simulink model "PubIfDecisionLSM_MDL"  (R2020b)
settings: configuration reference "DspaceConfig" (kept outside this file)
PostLoadFcn:
  | if any(exist('dsrtsu_mdlpostloadfcn', 'file') ~= 0), dsrtsu_mdlpostloadfcn('Execute', bdroot); end
InitFcn:
  | , if any(exist('rtifpga_mdlclblib', 'file') ~= 0), rtifpga_mdlclblib('Init', bdroot); end,
  | , if any(exist('dsmpb_private', 'file') ~= 0), dsmpb_private('dsmpb_mdlclblib', 'Init', bdroot); end,
values from neighbouring files (symbols this model uses):
  P_LSM_ALC_Enable = 0.0    [LSM_Parameter.sldd]
  P_LSM_AwayEdge_offset = 0.1    [LSM_Parameter.sldd]
  P_LSM_CentValidErr = 1.0    [LSM_Parameter.sldd]
  P_LSM_DOP_C0_EN_Limit = 0.8    [LSM_Parameter.sldd]
  P_LSM_DOP_C0_out_Limit = 2.0    [LSM_Parameter.sldd]
  P_LSM_DOP_C1_EN_Limit : value not decoded    [LSM_Parameter.sldd]
  P_LSM_DOP_C1_out_Limit : value not decoded    [LSM_Parameter.sldd]
  P_LSM_DOP_C1AndC2_Lim_X : value not decoded    [LSM_Parameter.sldd]
  P_LSM_DOP_C2_EN_Limit : value not decoded    [LSM_Parameter.sldd]
  P_LSM_DOP_C2_out_Limit : value not decoded    [LSM_Parameter.sldd]
  P_LSM_DOP_In_Pre2Dop_Dis = 1.0    [LSM_Parameter.sldd]
  P_LSM_DOP_Out_Pre2Dop_Dis = 2.0    [LSM_Parameter.sldd]
  P_LSM_DOP_PreDis_X : value not decoded    [LSM_Parameter.sldd]
  P_LSM_DOP_PreDis_Y : value not decoded    [LSM_Parameter.sldd]
  P_LSM_DOPEnableSW = 1.0    [LSM_Parameter.sldd]
  P_LSM_DOPValid_CheckTime = 0.06    [LSM_Parameter.sldd]
  P_LSM_DoubleLine_Curr2Cent_Dislimit = 0.5    [LSM_Parameter.sldd]
  P_LSM_DoubleLine_Dop2Cent_Dislimit = 0.5    [LSM_Parameter.sldd]
  P_LSM_DoubleLine_DOPOut_C1 : value not decoded    [LSM_Parameter.sldd]
  P_LSM_DoubleLine_Pre2Cent_Dislimit = 1.0    [LSM_Parameter.sldd]
  P_LSM_Error_Limit = 0.5    [LSM_Parameter.sldd]
  P_LSM_IFV2CenterAxis = 0.0    [LSM_Parameter.sldd]
  P_LSM_IFV2RearAxis = 0.0    [LSM_Parameter.sldd]
  P_LSM_Line2Edge_limit = 0.5    [LSM_Parameter.sldd]
  P_LSM_Line_Error = 0.1    [LSM_Parameter.sldd]
  P_LSM_LineSTD_Limit = 0.15    [LSM_Parameter.sldd]
  P_LSM_NOH_Switch = 0.0    [LSM_Parameter.sldd]
  P_LSM_OTL_C0_Factor = 1.0    [LSM_Parameter.sldd]
  P_LSM_OTL_C1_Factor = 0.5    [LSM_Parameter.sldd]
  P_LSM_OTL_C2_Factor = 0.5    [LSM_Parameter.sldd]
  P_LSM_Pre2OnlyLineDis = 5.0    [LSM_Parameter.sldd]
  P_LSM_Pre_t = 0.0    [LSM_Parameter.sldd]
  P_LSM_SingleLine_Cent2Edge_Dislimit = 100.0    [LSM_Parameter.sldd]
  P_LSM_SingleLine_Curr2Cent_Dislimit = 0.2    [LSM_Parameter.sldd]
  P_LSM_SingleLine_Dop2Cent_Dislimit = 0.2    [LSM_Parameter.sldd]
  P_LSM_SingleLine_DOPOut_C1 : value not decoded    [LSM_Parameter.sldd]
  P_LSM_SingleLine_Pre2Cent_Dislimit = 0.5    [LSM_Parameter.sldd]
  P_LSM_TJALimitSpd = 60.0    [LSM_Parameter.sldd]
undefined symbols (not defined in the file or in its folder): P_lCS_IFV2CenterAxis, P_LCS_IFV2RearAxis, P_LSM_EntryEdge_offset, P_LSM_EntryLnChngEnSwitch, P_LSM_EntryVanishDis, P_LSM_LinetLostTime, P_LSM_LineWijCal_C12, P_LSM_LineWijCal_C13, P_LSM_MapValid_ErrorSwitch, P_LSM_PosLineLcFac, P_LSM_SpdLim_Stub_Spd, P_LSM_SpdLim_StubLength, P_LSM_SpdTurnAlarm
libraries: simulink x324, TrueDurationTime x11
(part 7 of 25)

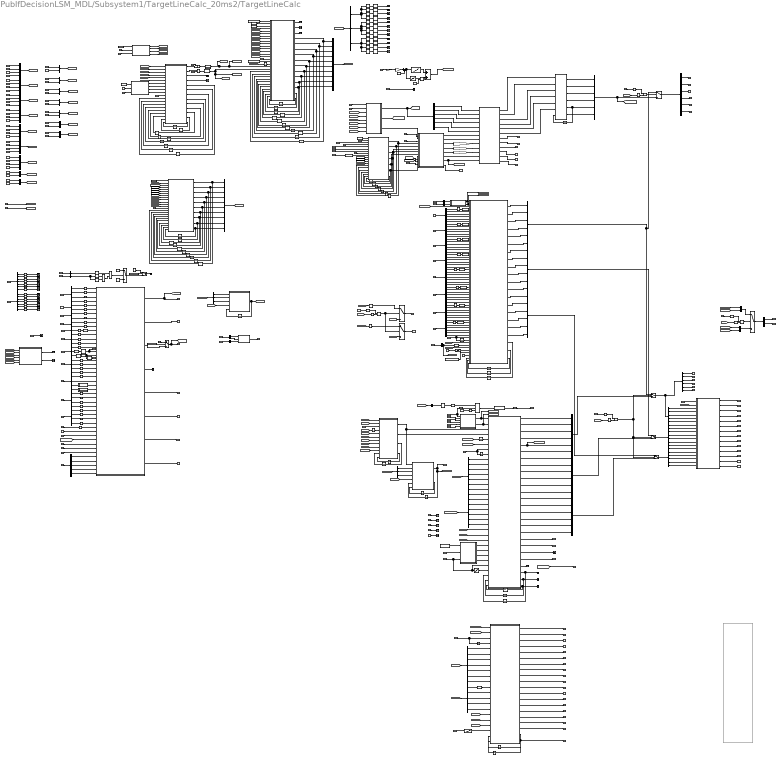
== system PubIfDecisionLSM_MDL/Subsystem1/TargetLineCalc_20ms2/TargetLineCalc ==
  kap : Inport
  vRef : Inport  Port=2
  OTLineValid : Inport  Port=3
  aOTL : Inport  Port=4
  bOTL : Inport  Port=5
  cOTL : Inport  Port=6
  dOTL : Inport  Port=7
  dxMax : Inport  Port=8
  OTLCount : Inport  Port=9
  ACCmode : Inport  Port=10
  HWASts : Inport  Port=11
  LRELineUpdate : Inport  Port=12
  LALineUpdate : Inport  Port=13
  LeftLine_Change : Inport  Port=14
  RightLine_Change : Inport  Port=15
  L1_Conf : Inport  Port=16
  L2_Conf : Inport  Port=17
  L3_Conf : Inport  Port=18
  L4_Conf : Inport  Port=19
  L1_A3 : Inport  Port=20
  L2_A3 : Inport  Port=21
  L3_A3 : Inport  Port=22
  L4_A3 : Inport  Port=23
  L1_A2 : Inport  Port=24
  L2_A2 : Inport  Port=25
  L3_A2 : Inport  Port=26
  L4_A2 : Inport  Port=27
  L1_A1 : Inport  Port=28
  L2_A1 : Inport  Port=29
  L3_A1 : Inport  Port=30
  L4_A1 : Inport  Port=31
  L1_A0 : Inport  Port=32
  L2_A0 : Inport  Port=33
  L3_A0 : Inport  Port=34
  L4_A0 : Inport  Port=35
  L1_R : Inport  Port=36
  L2_R : Inport  Port=37
  L3_R : Inport  Port=38
  L4_R : Inport  Port=39
  L1_Re : Inport  Port=40
  L2_Re : Inport  Port=41
  L3_Re : Inport  Port=42
  L4_Re : Inport  Port=43
  Edge1_R : Inport  Port=44
  Edge2_R : Inport  Port=45
  Edge1_A3 : Inport  Port=46
  Edge2_A3 : Inport  Port=47
  Edge1_A2 : Inport  Port=48
  Edge2_A2 : Inport  Port=49
  Edge1_A1 : Inport  Port=50
  Edge2_A1 : Inport  Port=51
  Edge1_A0 : Inport  Port=52
  Edge2_A0 : Inport  Port=53
  Edge1_Conf : Inport  Port=54
  Edge2_Conf : Inport  Port=55
  Edge1_Re : Inport  Port=56
  Edge2_Re : Inport  Port=57
  LeftLineType : Inport  Port=58
  RightLineType : Inport  Port=59
  LeftDLM : Inport  Port=60
  RightDLM : Inport  Port=61
  LH1Color : Inport  Port=62
  LH2Color : Inport  Port=63
  LeftDECEL : Inport  Port=64
  RightDECEL : Inport  Port=65
  pathPredValid : Inport  Port=66
  pathPredC3 : Inport  Port=67
  pathPredC2 : Inport  Port=68
  pathPredC1 : Inport  Port=69
  pathPredC0 : Inport  Port=70
  ESSSts : Inport  Port=71
  LCKSts : Inport  Port=72
  RFM_INTERSEC_ALERT : Inport  Port=73
  RFM_CURRENT_LANE : Inport  Port=74
  RFM_RIGHT_LANE : Inport  Port=75
  RFM_BRANCH : Inport  Port=76
  RFM_ROAD : Inport  Port=77  OutDataTypeStr=Bus: RFM_ROAD_BUS  PortDimensions=1  BusOutputAsStruct=on
  RFM_LINE_ENTRY_CL : Inport  Port=78
  RFM_LINE_EXIT_CL : Inport  Port=79
  RFM_LINE_CL : Inport  Port=80
  RFM_TSR_BUS : Inport  Port=81  OutDataTypeStr=Bus: RFM_TSR_BUS
  RFM_REC_LANES : Inport  Port=82
  RFM_LINE_L1 : Inport  Port=83
  RFM_LINE_R1 : Inport  Port=84
  RFM_LINE_L2 : Inport  Port=85
  RFM_LINE_R2 : Inport  Port=86
  RFM_LEFT_LANE : Inport  Port=87
  RFM_ODD : Inport  Port=88  OutDataTypeStr=Bus: RFM_ODD_BUS  PortDimensions=1  BusOutputAsStruct=on
  NOH_Sts : Inport  Port=89
  RFM_LINE_RB : Inport  Port=90
  AND{,1..3} (4 alike) : Logic  AllPortsSameDT=off  OutDataTypeStr=boolean
  Add : Sum
  Bus Creator : BusCreator  Inputs=10
  Bus Creator1 : BusCreator  Inputs=10
  Bus Creator10 : BusCreator  Inputs=2
  Bus Creator{2..8} (7 alike) : BusCreator  Inputs=6
  Bus Creator9 : BusCreator  Inputs=2
  Bus Selector : BusSelector  OutputSignals=LineConf,A1,A0
  Bus Selector1 : BusSelector  OutputSignals=LineConf
  Bus Selector{9..10,23,39} (4 alike) : BusSelector  OutputSignals=HWALineValid,HWALineC3,HWALineC2,HWALineC1,HWALineC0,HWARange
  Bus Selector11 : BusSelector  OutputSignals=HWALeLineValid,HWALeLineC3,HWALeLineC2,HWALeLineC1,HWALeLineC0,HWALeRange
  Bus Selector12 : BusSelector  OutputSignals=b_is_available,f_start_distance,f_end_distance,en_direction
  Bus Selector13 : BusSelector  OutputSignals=i_mapvalid
  Bus Selector14 : BusSelector  OutputSignals=nLaneNum,nLaneID
  Bus Selector15 : BusSelector  OutputSignals=b_vanish_valid
  Bus Selector{7,16,20..21,29} (5 alike) : BusSelector  OutputSignals=bIsLineExist,dC0V,dC1V,dC2V,dC3V,dDisFront
  Bus Selector17 : BusSelector  OutputSignals=dDisStart,bIsLineExist,dC0V
  Bus Selector18 : BusSelector  OutputSignals=bIsLineExist,dC0V,dC1V,dC2V,dC3V,dDisStart,dDisFront
  Bus Selector19 : BusSelector  OutputSignals=bIsLineExist,dC0V,dC1V,dC2V,dC3V,dDisStart,dDisFront
  Bus Selector2 : BusSelector  OutputSignals=LineConf,LineReliable,A3,A2,A1,A0,Range,tLost
  Bus Selector22 : BusSelector  OutputSignals=Avail_time,Avail_dis,A0
  Bus Selector24 : BusSelector  OutputSignals=RoadType
  Bus Selector25 : BusSelector  OutputSignals=b_is_avalible,en_lane_type,b_vanish_valid,f_vanish_pt_dis
  Bus Selector26 : BusSelector  OutputSignals=i_rec_lanes_num,i_rec_lanes
  Bus Selector27 : BusSelector  OutputSignals=eLineType
  Bus Selector28 : BusSelector  OutputSignals=eLineType
  Bus Selector3 : BusSelector  OutputSignals=LineConf,A3,A2,A1,A0,Range,tLost
  Bus Selector30 : BusSelector  OutputSignals=HWARiLineValid,HWARiLineC3,HWARiLineC2,HWARiLineC1,HWARiLineC0,HWARiRange
  Bus Selector31 : BusSelector  OutputSignals=RoadType,VehInLeftmostLane,VehInRightmostLane
  Bus Selector32 : BusSelector  OutputSignals=i_mapvalid,i_on_nav_path
  Bus Selector33 : BusSelector  OutputSignals=bIsLineExist,dDisStart,dC0V
  Bus Selector34 : BusSelector  OutputSignals=SPL_LaneChanged
  Bus Selector35 : BusSelector  OutputSignals=f_vanish_pt_dis,en_lane_type,b_is_avalible,f_spd_change_dis,i_change_spd_max
  Bus Selector36 : BusSelector  OutputSignals=b_is_avalible,en_lane_type
  Bus Selector37 : BusSelector  OutputSignals=b_is_avalible
  Bus Selector38 : BusSelector  OutputSignals=b_is_avalible,en_lane_type,b_vanish_valid,f_vanish_pt_dis
  Bus Selector4 : BusSelector  OutputSignals=EdgeConf,EdgeA3,EdgeA2,EdgeA1,EdgeA0
  Bus Selector40 : BusSelector  OutputSignals=LeftEn,RightEn
  Bus Selector41 : BusSelector  OutputSignals=bIsLineExist,dC3V,dC2V,dC1V,dC0V
  Bus Selector42 : BusSelector  OutputSignals=bIsLineExist,dC0V,dC1V,dC2V,dC3V,dDisFront,dDisStart
  Bus Selector43 : BusSelector  OutputSignals=bIsLineExist,dC0V,dC1V,dC2V,dC3V,dDisFront,dDisStart
  Bus Selector5 : BusSelector  OutputSignals=EdgeConf,EdgeA1,EdgeA0
  Bus Selector6 : BusSelector  OutputSignals=CentLineConf,CentLineC3,CentLineC2,CentLineC1,CentLineC0,CentLineRange
  Bus Selector8 : BusSelector  OutputSignals=bIsLineExist,dC0V,dC1V,dC2V,dC3V,dDisFront,dDisStart
  CalcEgoVehMove : MATLAB Function  TreatAsAtomicUnit=on
  CalcEgoVehMove1 : MATLAB Function  TreatAsAtomicUnit=on
  CalcEgoVehMove2 : MATLAB Function  TreatAsAtomicUnit=on
  CenLineCal1 : Subsystem
  Compare To Constant10 : simulink/Logic and Bit Operations/Compare To Constant  relop===  const=2  OutDataTypeStr=boolean
  Compare To Constant{6..7,11..12,19..21,29} (8 alike) : simulink/Logic and Bit Operations/Compare To Constant  relop=>  const=1  OutDataTypeStr=boolean
  Compare To Constant{2..3,13,17} (4 alike) : simulink/Logic and Bit Operations/Compare To Constant  relop=~=  const=0  OutDataTypeStr=boolean
  Compare To Constant{4..5,14,18} (4 alike) : simulink/Logic and Bit Operations/Compare To Constant  relop=>  const=2  OutDataTypeStr=boolean
  Compare To Constant15 : simulink/Logic and Bit Operations/Compare To Constant  relop===  const=2  OutDataTypeStr=boolean
  Compare To Constant16 : simulink/Logic and Bit Operations/Compare To Constant  relop===  const=1  OutDataTypeStr=boolean
  Compare To Constant8 : simulink/Logic and Bit Operations/Compare To Constant  relop=>  const=0  OutDataTypeStr=boolean
  Compare To Constant9 : simulink/Logic and Bit Operations/Compare To Constant  relop===  const=1  OutDataTypeStr=boolean
  Compare To Zero : simulink/Logic and Bit Operations/Compare To Zero  relop=>  OutDataTypeStr=boolean
  Compare To Constant1 : simulink/Logic and Bit Operations/Compare To Constant  relop===  const=0  OutDataTypeStr=boolean
  Compare To Constant59 : simulink/Logic and Bit Operations/Compare To Constant  relop=~=  const=2  OutDataTypeStr=boolean
  Compare To Constant60 : simulink/Logic and Bit Operations/Compare To Constant  relop=>=  const=150  OutDataTypeStr=boolean
  Constant{,2..4} (4 alike) : Constant  Value=0.02  OutDataTypeStr=single
  Constant1 : Constant  Value=P_LSM_LinetLostTime
  Constant10 : Constant  Value=P_LSM_NOH_Switch
  Constant11 : Constant  Value=P_LSM_EntryEdge_offset
  Constant14 : Constant  Value=P_LSM_LineSTD_Limit
  Constant15 : Constant  Value=0  OutDataTypeStr=uint8
  Constant16 : Constant  Value=3  OutDataTypeStr=uint8
  Constant17 : Constant  Value=0  OutDataTypeStr=uint8
  Constant18 : Constant  Value=P_LSM_ALC_Enable  OutDataTypeStr=uint8
  Constant6 : Constant  Value=0.05  OutDataTypeStr=single
  Constant7 : Constant  Value=P_LSM_Pre_t
  Constant8 : Constant  Value=1.3  OutDataTypeStr=single
  Constant9 : Constant  Value=2  OutDataTypeStr=uint8
  D : Lookup_n-D  NumberOfTableDimensions=1  BreakpointsForDimension1=[0,30,40]  Table=[15,25,25]  InternalRulePriority=Speed  RndMeth=Simplest  InputSameDT=on
  D1 : Lookup_n-D  NumberOfTableDimensions=1  BreakpointsForDimension1=[0,30,40]  Table=[10,25,25]  InternalRulePriority=Speed  RndMeth=Simplest  InputSameDT=on
  D2 : Lookup_n-D  NumberOfTableDimensions=1  BreakpointsForDimension1=[0,30,40]  Table=[15,25,25]  InternalRulePriority=Speed  RndMeth=Simplest  InputSameDT=on
  Data Type Conversion{,1..3} (4 alike) : DataTypeConversion  OutDataTypeStr=boolean
  Data Type Conversion{4..11} (8 alike) : DataTypeConversion
  Data Type Conversion12 : DataTypeConversion  OutDataTypeStr=uint8
  DetectChange : Subsystem
  DetectChange1 : Subsystem
  DetectIncrease : Subsystem
  DetectIncrease1 : Subsystem
  ESSLineCalc : MATLAB Function  Commented=on  TreatAsAtomicUnit=on
  ESSLineCalc1 : MATLAB Function  TreatAsAtomicUnit=on
  Gain1 : Gain  Gain=P_LSM_OTL_C2_Factor
  Gain2 : Gain  Gain=P_LSM_OTL_C1_Factor
  Gain3 : Gain  Gain=3.6
  Gain4 : Gain  Gain=1.03
  Gain5 : Gain  Gain=P_LSM_OTL_C0_Factor
  HWALineCalc : MATLAB Function  TreatAsAtomicUnit=on
  HWASts1 : InportShadow  Port=11
  HWASts2 : InportShadow  Port=11
  HWASts3 : InportShadow  Port=11
  LCKSts1 : InportShadow  Port=72
  LREWidthCalc : MATLAB Function  TreatAsAtomicUnit=on
  LeftLineType1 : InportShadow  Port=58
  LineSelect : MATLAB Function  TreatAsAtomicUnit=on
  Logical Operator : Logic  Inputs=3  AllPortsSameDT=off  OutDataTypeStr=boolean
  Logical Operator1 : Logic  Operator=OR  AllPortsSameDT=off  OutDataTypeStr=boolean
  Logical Operator2 : Logic  Operator=OR  AllPortsSameDT=off  OutDataTypeStr=boolean
  Logical Operator7 : Logic  AllPortsSameDT=off  OutDataTypeStr=boolean
  Logical Operator8 : Logic  Operator=OR  AllPortsSameDT=off  OutDataTypeStr=boolean
  MATLAB Function : MATLAB Function  TreatAsAtomicUnit=on
  MATLAB Function1 : MATLAB Function  TreatAsAtomicUnit=on
  Mux{,1..5,12} (7 alike) : Mux
  Mux{6..11,13..15} (9 alike) : Mux  Inputs=2
  NOA : MATLAB Function  TreatAsAtomicUnit=on
  NOH_Sts{1..4} (4 alike) : InportShadow  Port=89
  Product : Product
  RFM_CURRENT_LANE1 : InportShadow  Port=74
  RFM_CURRENT_LANE2 : InportShadow  Port=74
  RFM_LINE_ENTRY_CL1 : InportShadow  Port=78
  RFM_LINE_ENTRY_CL2 : InportShadow  Port=78
  RFM_LINE_ENTRY_CL3 : InportShadow  Port=78
  RFM_LINE_EXIT_CL1 : InportShadow  Port=79
  RFM_LINE_EXIT_CL2 : InportShadow  Port=79
  RFM_LINE_L3 : InportShadow  Port=83
  RFM_LINE_R3 : InportShadow  Port=84
  RFM_RIGHT_LANE1 : InportShadow  Port=75
  RFM_ROAD1 : InportShadow  Port=77  OutDataTypeStr=Bus: RFM_ROAD_BUS  PortDimensions=1  BusOutputAsStruct=on
  RFM_ROAD2 : InportShadow  Port=77  OutDataTypeStr=Bus: RFM_ROAD_BUS  PortDimensions=1  BusOutputAsStruct=on
  RFM_TSR_BUS1 : InportShadow  Port=81  OutDataTypeStr=Bus: RFM_TSR_BUS
  RFM_TSR_BUS2 : InportShadow  Port=81  OutDataTypeStr=Bus: RFM_TSR_BUS
  RightLineType1 : InportShadow  Port=59
  RoadWidthCalc1 : MATLAB Function  TreatAsAtomicUnit=on
  Selector : Selector  InputPortWidth=4  IndexOptions=Index vector (dialog)  Indices=2  OutputSizes=1
  Selector{1,4..5,10} (4 alike) : Selector  InputPortWidth=4  IndexOptions=Index vector (dialog)  Indices=1  OutputSizes=1
  Selector11 : Selector  InputPortWidth=4  IndexOptions=Index vector (dialog)  Indices=4  OutputSizes=1
  Selector12 : Selector  InputPortWidth=4  IndexOptions=Index vector (dialog)  Indices=3  OutputSizes=1
  Selector2 : Selector  InputPortWidth=4  IndexOptions=Index vector (dialog)  Indices=3  OutputSizes=1
  Selector3 : Selector  InputPortWidth=4  IndexOptions=Index vector (dialog)  Indices=2  OutputSizes=1
  Selector6 : Selector  InputPortWidth=4  IndexOptions=Index vector (dialog)  Indices=4  OutputSizes=1
  Selector7 : Selector  InputPortWidth=4  IndexOptions=Index vector (dialog)  Indices=4  OutputSizes=1
  Selector8 : Selector  InputPortWidth=4  IndexOptions=Index vector (dialog)  Indices=3  OutputSizes=1
  Selector9 : Selector  InputPortWidth=4  IndexOptions=Index vector (dialog)  Indices=2  OutputSizes=1
  Signal Copy{,1..42,44..57} (57 alike) : SignalConversion  OverrideOpt=off
  Subsystem : Subsystem
  Subsystem1 : Subsystem
  Subsystem2 : Subsystem
  Subsystem3 : Subsystem
  Sum : Sum  Inputs=|++
  Switch{,1..9} (10 alike) : Switch  Criteria=u2 > Threshold
  TJA2NOA : MATLAB Function  TreatAsAtomicUnit=on
  Terminator{,1..46} (47 alike) : Terminator
  Tracker : MATLAB Function  TreatAsAtomicUnit=on
  TrueDurationTime : TrueDurationTime/TrueDurationTime  TCycle=0.02
  TypeConf : Subsystem
  TypeConf1 : Subsystem
  Unit Delay{,1,3,6,10..13,15,27,30,32,34..35,39..41,49,58..59,64} (21 alike) : UnitDelay  SampleTime=-1  HasFrameUpgradeWarning=on
  Unit Delay14 : UnitDelay  InitialCondition=3.75  SampleTime=-1  HasFrameUpgradeWarning=on
  Unit Delay16 : UnitDelay  InitialCondition=uint8(0)  SampleTime=-1  HasFrameUpgradeWarning=on
  Unit Delay{17..22,38} (7 alike) : UnitDelay  InitialCondition=single(zeros(2,1))  SampleTime=-1  HasFrameUpgradeWarning=on
  Unit Delay2 : UnitDelay  InitialCondition=[5;5;5;5]  SampleTime=-1  HasFrameUpgradeWarning=on
  Unit Delay23 : UnitDelay  InitialCondition=uint8(zeros(2,1))  SampleTime=-1  HasFrameUpgradeWarning=on
  Unit Delay24 : UnitDelay  InitialCondition=uint8(0)  SampleTime=-1  HasFrameUpgradeWarning=on
  Unit Delay25 : UnitDelay  InitialCondition=false  SampleTime=-1  HasFrameUpgradeWarning=on
  Unit Delay26 : UnitDelay  InitialCondition=int8(0)  SampleTime=-1  HasFrameUpgradeWarning=on
  Unit Delay{4..5,7..9,28..29,37,57,60..61} (11 alike) : UnitDelay  InitialCondition=zeros(4,1)  SampleTime=-1  HasFrameUpgradeWarning=on
  Unit Delay33 : UnitDelay  InitialCondition=3.75  SampleTime=-1  HasFrameUpgradeWarning=on
  Unit Delay36 : UnitDelay  InitialCondition=8  SampleTime=-1  HasFrameUpgradeWarning=on
  Unit Delay42 : UnitDelay  InitialCondition=false  SampleTime=-1  HasFrameUpgradeWarning=on
  Unit Delay{43..48} (6 alike) : UnitDelay  InitialCondition=single(0)  SampleTime=-1  HasFrameUpgradeWarning=on
  Unit Delay62 : UnitDelay  InitialCondition=zeros(2,1)  SampleTime=-1  HasFrameUpgradeWarning=on
  Unit Delay63 : UnitDelay  InitialCondition=zeros(2,1)  SampleTime=-1  HasFrameUpgradeWarning=on
  Unit Delay65 : UnitDelay  InitialCondition=int8(0)  SampleTime=-1  HasFrameUpgradeWarning=on
  VehStation : MATLAB Function  TreatAsAtomicUnit=on
  VisLineFilter1 : MATLAB Function  TreatAsAtomicUnit=on
  VisLineFilter2 : MATLAB Function  TreatAsAtomicUnit=on
  VisLineFilter4 : MATLAB Function  TreatAsAtomicUnit=on
  YBranchRi : MATLAB Function  TreatAsAtomicUnit=on
  kap{1..6} (6 alike) : InportShadow
  preDisMinTable : Lookup_n-D  NumberOfTableDimensions=1  BreakpointsForDimension1=[0 5 10 15 20 25 30 35 40 60 80 90 100 110 120 140]  Table=[8 9 10 11 12 13 14 15 17 22 28 31 35 38 42 49]  ExtrapMethod=Clip  InternalRulePriority=Speed  RndMeth=Simplest  InputSameDT=on
  tDeltaEpsTable : Lookup_n-D  NumberOfTableDimensions=1  BreakpointsForDimension1=[0 5 10 15 20 25 30 35 40 60 80 90 100 110 120 140]  Table=[0.8 0.8 0.77803 0.75258 0.71864 0.65924 0.5447 0.45773 0.38348 0.2 0.2 0.2 0.20106 0.2 0.2 0.2]  ExtrapMethod=Clip  InternalRulePriority=Speed  RndMeth=Simplest  InputSameDT=on
  tFilt : Constant  Value=0.2  OutDataTypeStr=single
  vRef{1,3..16} (15 alike) : InportShadow  Port=2
  TJALineValid : Outport
  TJALineA3 : Outport  Port=2
  TJALineA2 : Outport  Port=3
  TJALineA1 : Outport  Port=4
  TJALineA0 : Outport  Port=5
  TJALineRange : Outport  Port=6
  LCKLineValid : Outport  Port=7
  LCKLineA3 : Outport  Port=8
  LCKLineA2 : Outport  Port=9
  LCKLineA1 : Outport  Port=10
  LCKLineA0 : Outport  Port=11
  LCKLineRange : Outport  Port=12
  HWALineValid : Outport  Port=13
  HWALineA3 : Outport  Port=14
  HWALineA2 : Outport  Port=15
  HWALineA1 : Outport  Port=16
  HWALineA0 : Outport  Port=17
  HWALineRange : Outport  Port=18
  HWALineLValid : Outport  Port=19
  HWALineLA3 : Outport  Port=20
  HWALineLA2 : Outport  Port=21
  HWALineLA1 : Outport  Port=22
  HWALineLA0 : Outport  Port=23
  HWALineLRange : Outport  Port=24
  HWALineRValid : Outport  Port=25
  HWALineRA3 : Outport  Port=26
  HWALineRA2 : Outport  Port=27
  HWALineRA1 : Outport  Port=28
  HWALineRA0 : Outport  Port=29
  HWALineRRange : Outport  Port=30
  pre_dy_Error : Outport  Port=31
  pre_HeadAng_Error : Outport  Port=32
  MLeLane : Outport  Port=33
  RoadWidth : Outport  Port=34
  SingleLineLost_b : Outport  Port=35
  DoubleLineLost_b : Outport  Port=36
  LeLineCrossing : Outport  Port=37
  RiLineCrossing : Outport  Port=38
  MRiLane : Outport  Port=39
  MrcStopLane : Outport  Port=40
  ESSLineValid : Outport  Port=41
  ESSLineA3 : Outport  Port=42
  ESSLineA2 : Outport  Port=43
  ESSLineA1 : Outport  Port=44
  ESSLineA0 : Outport  Port=45
  ESSLineRange : Outport  Port=46
  ESSLineLValid : Outport  Port=47
  ESSLineLA3 : Outport  Port=48
  ESSLineLA2 : Outport  Port=49
  ESSLineLA1 : Outport  Port=50
  ESSLineLA0 : Outport  Port=51
  ESSLineLRange : Outport  Port=52
  ESSLineRValid : Outport  Port=53
  ESSLineRA3 : Outport  Port=54
  ESSLineRA2 : Outport  Port=55
  ESSLineRA1 : Outport  Port=56
  ESSLineRA0 : Outport  Port=57
  ESSLineRRange : Outport  Port=58
  ESSLineLock_b : Outport  Port=59
  leftLaneCurise_b : Outport  Port=60
  PilotSts : Outport  Port=61
  PilotTurnSwSts : Outport  Port=62
  PilotSPLDist : Outport  Port=63
  PilotSPL : Outport  Port=64
  TJALineSource : Outport  Port=65
  PilotRoadSts : Outport  Port=66
  LSM_PilotNohExitDist : Outport  Port=67
  LSM_HMI_Voice : Outport  Port=68
  LeLineLcAvailable : Outport  Port=69
  RiLineLcAvailable : Outport  Port=70
  LeLineVirtual_b : Outport  Port=71
  RiLineVirtual_b : Outport  Port=72
  tag scope: RoadWidth=global, VisEdge=global, VisLine=global
  wires:
  Gain5/1 -> LineSelect/11(dOTL)
  Gain2/1 -> LineSelect/10(cOTL)
  Gain1/1 -> LineSelect/9(bOTL)
  Data Type Conversion12/1 -> MRiLane/1
  Data Type Conversion3/1 -> Subsystem3/17(VehInRightmostLane), Data Type Conversion12/1
  Signal Copy/1 -> Data Type Conversion3/1
  kap1/1 -> Subsystem2/12(kap)
  [VisEdge] -> Subsystem2/11(EdgeLine)
  [CentLine] -> Subsystem2/10(CentLine)
  Subsystem1/1(Out1) -> Subsystem3/24(ChgSpd_Dis)
  Subsystem/1(Out1) -> Subsystem3/25(SpdChgMax)
  Bus Selector35/5 -> Subsystem/1(Spd)  "<i_change_spd_max>"
  Bus Selector35/4 -> Subsystem1/1(Dis)  "<f_spd_change_dis>"
  kap6/1 -> NOA/62(kap)
  Constant11/1 -> NOA/61(Offset)
  Unit Delay/1 -> NOA/64(LockIDK1)
  Data Type Conversion11/1 -> NOA/42(LineRB_Valid)
  Compare To Constant21/1 -> Data Type Conversion11/1
  Bus Selector43/7 -> NOA/48(LineRB_Start)  "<dDisStart>"
  Bus Selector43/6 -> NOA/47(LineRB_Range)  "<dDisFront>"
  Bus Selector43/5 -> NOA/46(LineRB_A3)  "<dC3V>"
  Bus Selector43/4 -> NOA/45(LineRB_A2)  "<dC2V>"
  Bus Selector43/3 -> NOA/44(LineRB_A1)  "<dC1V>"
  Bus Selector43/2 -> NOA/43(LineRB_A0)  "<dC0V>"
  Bus Selector43/1 -> Compare To Constant21/1  "<bIsLineExist>"
  RFM_LINE_RB/1 -> Bus Selector43/1
  Bus Selector42/7 -> NOA/41(Entry_Start)  "<dDisStart>"
  Bus Selector42/6 -> NOA/40(Entry_Range)  "<dDisFront>"
  Bus Selector42/5 -> NOA/39(Entry_A3)  "<dC3V>"
  Bus Selector42/4 -> NOA/38(Entry_A2)  "<dC2V>"
  Bus Selector42/3 -> NOA/37(Entry_A1)  "<dC1V>"
  Bus Selector42/2 -> NOA/36(Entry_A0)  "<dC0V>"
  Data Type Conversion10/1 -> NOA/35(Entry_Valid)
  Bus Selector42/1 -> Compare To Constant20/1  "<bIsLineExist>"
  Compare To Constant20/1 -> Data Type Conversion10/1
  RFM_LINE_ENTRY_CL3/1 -> Bus Selector42/1
  Bus Selector41/5 -> Subsystem3/45(TarLineA0)  "<dC0V>"
  Bus Selector41/4 -> Subsystem3/44(TarLineA1)  "<dC1V>"
  Bus Selector41/3 -> Subsystem3/43(TarLineA2)  "<dC2V>"
  Bus Selector41/2 -> Subsystem3/42(TarLineA3)  "<dC3V>"
  Bus Selector41/1 -> Subsystem3/41(TarLineValid)  "<bIsLineExist>"
  RFM_LINE_ENTRY_CL2/1 -> Bus Selector41/1
  vRef16/1 -> Subsystem3/40(VxvRef)
  kap5/1 -> Subsystem3/39(KapTraj)
  HWASts3/1 -> Subsystem3/38(HWASts)
  RightDECEL/1 -> TypeConf/6(RightDECELType)
  LeftDECEL/1 -> TypeConf/3(LeftDECELType)
  Bus Selector35/3 -> Subsystem3/23(currentLane_valid)  "<b_is_avalible>"
  Data Type Conversion8/1 -> NOA/49(RFM_LineCL_Valid)
  Compare To Constant12/1 -> Data Type Conversion8/1
  Data Type Conversion7/1 -> NOA/22(RFM_LineR2_Valid)
  Data Type Conversion6/1 -> NOA/16(RFM_LineR1_Valid)
  Data Type Conversion5/1 -> NOA/10(RFM_LineL2_Valid)
  Data Type Conversion4/1 -> NOA/4(RFM_LineL1_Valid)
  Compare To Constant11/1 -> Data Type Conversion7/1
  Compare To Constant7/1 -> Data Type Conversion5/1
  Compare To Constant6/1 -> Data Type Conversion6/1
  Compare To Constant29/1 -> Data Type Conversion4/1
  vRef15/1 -> Subsystem3/36(vehSpd)
  Bus Selector35/2 -> Signal Copy48/1  "<en_lane_type>"
  Bus Selector38/2 -> Signal Copy50/1  "<en_lane_type>"
  Bus Selector25/2 -> Signal Copy52/1  "<en_lane_type>"
  [PilotSts] -> Compare To Constant2/1
  Compare To Constant2/1 -> AND1/2
  Compare To Constant5/1 -> AND1/1
  NOH_Sts2/1 -> Compare To Constant5/1
  AND/1 -> Switch1/2
  Compare To Constant4/1 -> AND/1
  NOH_Sts/1 -> Compare To Constant4/1
  Subsystem3/8(NOH_HMI_Voice) -> LSM_HMI_Voice/1  "LSM_HMI_Voice"
  Constant1/1 -> VisLineFilter2/1(P_LSM_LinetLostTime)
  Subsystem3/7(LSM_PilotNohExitDist) -> LSM_PilotNohExitDist/1  "LSM_PilotNohExitDist"
  RFM_ODD/1 -> Signal Copy53/1
  [LeftOffset_b] -> CenLineCal1/7(LeftLane_change)
  [RightOffset_b] -> CenLineCal1/8(RightLane_change)
  Bus Selector38/1 -> Signal Copy49/1  "<b_is_avalible>"
  RFM_RIGHT_LANE1/1 -> Bus Selector38/1
  Bus Selector25/1 -> Signal Copy51/1  "<b_is_avalible>"
  RFM_LEFT_LANE/1 -> Bus Selector25/1
  MATLAB Function/1(MrcStopLane) -> MrcStopLane/1
  Bus Selector36/1 -> MATLAB Function/1(Cur_avail)  "<b_is_avalible>"
  Bus Selector36/2 -> MATLAB Function/2(Cur_LaneType)  "<en_lane_type>"
  RFM_RIGHT_LANE/1 -> Bus Selector37/1
  RFM_CURRENT_LANE2/1 -> Bus Selector36/1
  Bus Selector37/1 -> MATLAB Function/3(Right_avail)  "<b_is_avalible>"
  DetectChange1/1(Out1) -> NOA/58(LaneChange)
  RFM_CURRENT_LANE1/1 -> Bus Selector35/1
  Bus Selector35/1 -> Signal Copy47/1  "<f_vanish_pt_dis>"
  Data Type Conversion2/1 -> Signal Copy8/1
  Data Type Conversion/1 -> Subsystem3/11(curr_b_vanish_valid)
  RFM_TSR_BUS2/1 -> Bus Selector34/1
  VehStation/2(RightMostLane) -> Terminator46/1
  VehStation/1(LeftMostLane) -> Terminator45/1
  Bus Selector31/2 -> Data Type Conversion2/1  "<VehInLeftmostLane>"
  Bus Selector33/3 -> Signal Copy46/1  "<dC0V>"
  Bus Selector33/2 -> Signal Copy45/1  "<dDisStart>"
  Bus Selector33/1 -> Signal Copy44/1  "<bIsLineExist>"
  RFM_LINE_ENTRY_CL1/1 -> Bus Selector33/1
  Bus Selector31/3 -> Signal Copy/1  "<VehInRightmostLane>"
  Bus Selector31/1 -> Signal Copy42/1  "<RoadType>"
  Bus Selector17/3 -> Signal Copy41/1  "<dC0V>"
  Bus Selector17/2 -> Signal Copy40/1  "<bIsLineExist>"
  Bus Selector17/1 -> Signal Copy39/1  "<dDisStart>"
  Bus Selector32/2 -> Signal Copy36/1  "<i_on_nav_path>"
  Bus Selector32/1 -> Signal Copy9/1  "<i_mapvalid>"
  Unit Delay49/1 -> TJA2NOA/7(HWALineC0K1)
  RFM_ROAD2/1 -> Bus Selector32/1
  RFM_TSR_BUS1/1 -> Bus Selector31/1
  Compare To Constant3/1 -> AND/2
  Bus Selector30/6 -> MATLAB Function1/20(RiLineRange)  "<HWARiRange>"
  Bus Selector30/5 -> MATLAB Function1/19(RiLineC0)  "<HWARiLineC0>"
  Bus Selector30/4 -> MATLAB Function1/18(RiLineC1)  "<HWARiLineC1>"
  Bus Selector30/3 -> MATLAB Function1/17(RiLineC2)  "<HWARiLineC2>"
  Bus Selector30/2 -> MATLAB Function1/16(RiLineC3)  "<HWARiLineC3>"
  Bus Selector30/1 -> MATLAB Function1/15(RiLineValid)  "<HWARiLineValid>"
  Switch3/1 -> Bus Selector30/1
  Bus Creator8/1 -> Switch3/1
  Bus Creator7/1 -> Switch3/3
  Bus Creator6/1 -> Switch2/1
  Bus Creator5/1 -> Switch1/1, Switch/1
  NOA/9(HWALeLineC2) -> Bus Creator6/3
  Bus Selector7/4 -> NOA/13(RFM_LineL2_A2)  "<dC2V>"
  Bus Selector29/5 -> NOA/8(RFM_LineL1_A3)  "<dC3V>"
  Bus Selector29/4 -> NOA/7(RFM_LineL1_A2)  "<dC2V>"
  NOA/13(HWARiLineValid) -> Bus Creator8/1
  NOA/6(HWARange) -> Bus Creator5/6
  NOA/10(HWALeLineC1) -> Bus Creator6/4
  NOA/2(HWALineC3) -> Bus Creator5/2
  NOA/18(HWARiRange) -> Bus Creator8/6
  [PilotRoadSts] -> NOA/59(PilotRoadSts)
  Bus Selector21/2 -> NOA/23(RFM_LineR2_A0)  "<dC0V>"
  NOA/12(HWALeRange) -> Bus Creator6/6
  Bus Selector7/2 -> NOA/11(RFM_LineL2_A0)  "<dC0V>"
  vRef8/1 -> D2/1
  Bus Selector7/1 -> Compare To Constant7/1  "<bIsLineExist>"
  Bus Selector20/5 -> NOA/20(RFM_LineR1_A3)  "<dC3V>"
  NOA/3(HWALineC2) -> Bus Creator5/3
  NOA/1(HWALineValid) -> Bus Creator5/1
  Bus Selector7/5 -> NOA/14(RFM_LineL2_A3)  "<dC3V>"
  NOA/8(HWALeLineC3) -> Bus Creator6/2
  Bus Selector29/3 -> NOA/6(RFM_LineL1_A1)  "<dC1V>"
  TypeConf1/1(LeftEn) -> NOA/1(LeftEn), [RFM_LeLineLcAvailable]
  [PilotSts] -> NOA/57(PilotSts)
  Bus Selector16/3 -> NOA/51(RFM_LineCL_A1)  "<dC1V>"
  NOA/11(HWALeLineC0) -> Bus Creator6/5
  D2/1 -> NOA/60(DistanceLim)
  Unit Delay40/1 -> NOA/63(MoveIDK1)
  NOA/14(HWARiLineC3) -> Bus Creator8/2
  NOA/20(LockID) -> Unit Delay/1
  Bus Selector20/2 -> NOA/17(RFM_LineR1_A0)  "<dC0V>"
  NOA/19(MoveID) -> Unit Delay40/1
  NOA/16(HWARiLineC1) -> Bus Creator8/4
  Bus Selector16/6 -> NOA/54(RFM_LineCL_Range)  "<dDisFront>"
  Bus Selector29/6 -> NOA/9(RFM_LineL1_Range)  "<dDisFront>"
  Unit Delay39/1 -> NOA/56(HWAStsK1)
  Bus Selector21/3 -> NOA/24(RFM_LineR2_A1)  "<dC1V>"
  Bus Selector29/1 -> Compare To Constant29/1  "<bIsLineExist>"
  NOA/7(HWALeLineValid) -> Bus Creator6/1
  HWASts1/1 -> NOA/55(HWASts), Unit Delay39/1
  RFM_LINE_L2/1 -> Bus Selector7/1
  Bus Selector29/2 -> NOA/5(RFM_LineL1_A0)  "<dC0V>"
  Bus Selector16/1 -> Compare To Constant12/1  "<bIsLineExist>"
  RFM_LINE_EXIT_CL2/1 -> Bus Selector8/1
  Bus Selector20/3 -> NOA/18(RFM_LineR1_A1)  "<dC1V>"
  Bus Selector8/6 -> NOA/33(Exit_Range)  "<dDisFront>"
  Bus Selector21/1 -> Compare To Constant11/1  "<bIsLineExist>"
  Bus Selector21/4 -> NOA/25(RFM_LineR2_A2)  "<dC2V>"
  Bus Selector7/6 -> NOA/15(RFM_LineL2_Range)  "<dDisFront>"
  Bus Selector20/6 -> NOA/21(RFM_LineR1_Range)  "<dDisFront>"
  NOA/15(HWARiLineC2) -> Bus Creator8/3
  Bus Selector8/2 -> NOA/29(Exit_A0)  "<dC0V>"
  Bus Selector16/4 -> NOA/52(RFM_LineCL_A2)  "<dC2V>"
  Bus Selector8/3 -> NOA/30(Exit_A1)  "<dC1V>"
  RFM_LINE_R2/1 -> Bus Selector21/1
  Bus Selector21/5 -> NOA/26(RFM_LineR2_A3)  "<dC3V>"
  TypeConf1/2(RightEn) -> NOA/2(RightEn), [RFM_RiLineLcAvailable]
  Bus Selector16/2 -> NOA/50(RFM_LineCL_A0)  "<dC0V>"
  NOA/17(HWARiLineC0) -> Bus Creator8/5
  Bus Selector8/4 -> NOA/31(Exit_A2)  "<dC2V>"
  Bus Selector8/1 -> Compare To Constant19/1  "<bIsLineExist>"
  RFM_LINE_L3/1 -> Bus Selector29/1
  Bus Selector27/1 -> TypeConf1/1(LeftType)  "<eLineType>"
  Bus Selector20/4 -> NOA/19(RFM_LineR1_A2)  "<dC2V>"
  NOA/5(HWALineC0) -> Bus Creator5/5
  RFM_LINE_L1/1 -> Bus Selector27/1
  NOA/4(HWALineC1) -> Bus Creator5/4
  Bus Selector34/1 -> [SPL_LaneChanged], DetectChange1/1(In1)  "<SPL_LaneChanged>"
  Bus Selector8/5 -> NOA/32(Exit_A3)  "<dC3V>"
  RFM_LINE_R1/1 -> Bus Selector28/1
  Bus Selector20/1 -> Compare To Constant6/1  "<bIsLineExist>"
  NOA/21(Lock_counter) -> Unit Delay41/1
  RFM_LINE_R3/1 -> Bus Selector20/1
  RFM_LINE_CL/1 -> Bus Selector16/1
  Unit Delay41/1 -> NOA/65(Lock_counterK1)
  Bus Selector28/1 -> TypeConf1/2(RightType)  "<eLineType>"
  Bus Selector7/3 -> NOA/12(RFM_LineL2_A1)  "<dC1V>"
  Bus Selector21/6 -> NOA/27(RFM_LineR2_Range)  "<dDisFront>"
  Bus Selector16/5 -> NOA/53(RFM_LineCL_A3)  "<dC3V>"
  Bus Selector8/7 -> NOA/34(Exit_Start)  "<dDisStart>"
  Subsystem3/4(LaneChange) -> Terminator44/1
  RFM_BRANCH/1 -> Terminator43/1
  Bus Selector15/1 -> Signal Copy37/1  "<b_vanish_valid>"
  RFM_CURRENT_LANE/1 -> Bus Selector15/1
  Bus Selector14/2 -> Signal Copy7/1  "<nLaneID>"
  Bus Selector14/1 -> Signal Copy6/1  "<nLaneNum>"
  RFM_ROAD1/1 -> Bus Selector14/1
  Bus Selector26/2 -> Signal Copy5/1  "<i_rec_lanes>"
  Bus Selector26/1 -> Signal Copy4/1  "<i_rec_lanes_num>"
  RFM_REC_LANES/1 -> Bus Selector26/1
  Constant18/1 -> Switch6/2
  Constant17/1 -> Switch6/1
  Switch6/1 -> Terminator42/1
  RFM_TSR_BUS/1 -> Bus Selector24/1
  Bus Selector13/1 -> Compare To Constant8/1  "<i_mapvalid>"
  Constant16/1 -> Switch5/3
  Logical Operator8/1 -> Logical Operator7/2
  Switch5/1 -> Switch6/3
  Constant15/1 -> Switch5/1
  Logical Operator7/1 -> Switch5/2
  Compare To Constant10/1 -> Logical Operator8/2
  Compare To Constant9/1 -> Logical Operator8/1
  Bus Selector24/1 -> Compare To Constant9/1, Compare To Constant10/1  "<RoadType>"
  Compare To Constant8/1 -> Logical Operator7/1
  Bus Selector23/6 -> HWALineCalc/22(PathPredRange)  "<HWARange>"
  Bus Selector23/5 -> HWALineCalc/21(PathPredA0)  "<HWALineC0>"
  Bus Selector23/1 -> HWALineCalc/17(PathPredValid)  "<HWALineValid>"
  Bus Selector23/4 -> HWALineCalc/20(PathPredA1)  "<HWALineC1>"
  Bus Selector23/2 -> HWALineCalc/18(PathPredA3)  "<HWALineC3>"
  Bus Selector23/3 -> HWALineCalc/19(PathPredA2)  "<HWALineC2>"
  [TJA_Line] -> Bus Selector23/1
  pathPredC0/1 -> Terminator40/1
  pathPredC1/1 -> Terminator39/1
  pathPredC2/1 -> Terminator38/1
  pathPredC3/1 -> Terminator37/1
  pathPredValid/1 -> Terminator36/1
  [Double_Line_Lost] -> DoubleLineLost_b/1  "DoubleLineLost_b"
  CenLineCal1/2(Double_Line_Lost) -> [Double_Line_Lost]
  [VisLineColor] -> VehStation/6(VisLineColor)
  Mux15/1 -> [VisLineColor]
  LH2Color/1 -> Mux15/2
  LH1Color/1 -> Mux15/1
  Constant10/1 -> Switch4/2
  Constant9/1 -> Switch4/1
  Switch4/1 -> PilotSts/1, [PilotSts]
  LCKSts1/1 -> Subsystem2/1(LCKSts)
  LCKSts/1 -> CenLineCal1/1(LCKSts)
  kap2/1 -> CenLineCal1/2(kap)
  [TJA_Line_State] -> HWALineCalc/6(TJA_Line_State)
  Subsystem2/7(TJA_Line_State) -> LineSelect/13(TJA_Line_State), [TJA_Line_State]  "LSM_TJA_Line_State"
  CenLineCal1/3(Line_State) -> Subsystem2/2(Line_State)
  vRef14/1 -> VisLineFilter1/2(vRef)
  [RoadWidth] -> CenLineCal1/6(RoadWidth)
  Product/1 -> Add/2
  vRef13/1 -> Product/2
  dOTL/1 -> VisLineFilter1/7(dOTL)
  cOTL/1 -> VisLineFilter1/6(cOTL)
  bOTL/1 -> VisLineFilter1/5(bOTL)
  Add/1 -> [preDis]
  tDeltaEpsTable/1 -> Product/1
  preDisMinTable/1 -> Add/1
  Sum/1 -> preDisMinTable/1, tDeltaEpsTable/1
  Gain3/1 -> Gain4/1
  Gain4/1 -> Sum/1
  Constant8/1 -> Sum/2
  vRef11/1 -> Gain3/1
  Subsystem2/8(Line_source) -> TJALineSource/1  "LSM_Line_source"
  Unit Delay29/1 -> VisLineFilter2/32(FaultK1)
  Unit Delay28/1 -> VisLineFilter2/31(fix_timeK1)
  VisLineFilter2/14(fix_time) -> Unit Delay28/1
  VisLineFilter2/15(Fault) -> Unit Delay29/1
  Bus Selector2/2 -> HWALineCalc/10(Reliable)  "<LineReliable>"
  [preDis] -> CenLineCal1/3(preDis)
  vRef10/1 -> Subsystem2/3(vRef)
  Subsystem2/6(OTL_Range) -> LineSelect/12(dxMax)
  Subsystem2/5(OTL_C0) -> Gain5/1
  Subsystem2/4(OTL_C1) -> Gain2/1
  Subsystem2/3(OTL_C2) -> Gain1/1
  Subsystem2/2(OTL_C3) -> LineSelect/8(aOTL)
  Subsystem2/1(OTL_Valid) -> LineSelect/7(OTLineValid)
  [VisLineReliable] -> YBranchRi/10(Reliable)
  Unit Delay27/1 -> HWALineCalc/5(HWALineC0K1)
  [HWALineC0] -> Unit Delay27/1
  [RightLineTypeEN] -> ESSLineCalc1/2(RightLineTypeEn)
  [LeftLineTypeEN] -> ESSLineCalc1/1(LeftLineTypeEn)
  Logical Operator1/1 -> DetectIncrease/1(In)
  DetectIncrease/1(Out) -> [LeLineCrossing], VisLineFilter2/19(LeftLineChange), [LeftOffset_b]
  Logical Operator2/1 -> DetectIncrease1/1(In)
  Bus Selector22/3 -> Selector10/1, Selector9/1, Selector11/1, Selector12/1  "<A0>"
  Selector10/1 -> Signal Copy32/1
  Selector9/1 -> Signal Copy33/1
  Signal Copy32/1 -> Terminator31/1  "LSM_L1_A0"
  Signal Copy33/1 -> Terminator32/1  "LSM_L2_A0"
  Signal Copy35/1 -> Terminator34/1  "LSM_L4_A0"
  Signal Copy34/1 -> Terminator33/1  "LSM_L3_A0"
  Selector11/1 -> Signal Copy35/1
  Selector12/1 -> Signal Copy34/1
  Selector8/1 -> Signal Copy30/1
  Selector7/1 -> Signal Copy31/1
  Signal Copy30/1 -> Terminator26/1  "LSM_L3_AvaliDis"
  Signal Copy31/1 -> Terminator27/1  "LSM_L4_AvaliDis"
  Selector6/1 -> Signal Copy29/1
  Signal Copy29/1 -> Terminator25/1  "LSM_L4_AvaliTime"
  Bus Selector22/1 -> Selector6/1, Selector2/1, Selector/1, Selector5/1  "<Avail_time>"
  Selector5/1 -> Signal Copy28/1
  Signal Copy28/1 -> Terminator24/1  "LSM_L1_AvaliTime"
  Signal Copy27/1 -> Terminator23/1  "LSM_L2_AvaliDis"
  Signal Copy26/1 -> Terminator22/1  "LSM_L1_AvaliDis"
  Signal Copy24/1 -> Terminator21/1  "LSM_L3_AvaliTime"
  Signal Copy25/1 -> Terminator20/1  "LSM_L2_AvaliTime"
  Selector3/1 -> Signal Copy27/1
  Selector4/1 -> Signal Copy26/1
  Bus Selector22/2 -> Selector8/1, Selector7/1, Selector3/1, Selector4/1  "<Avail_dis>"
  Selector2/1 -> Signal Copy24/1
  Selector/1 -> Signal Copy25/1
  [VisLine] -> Bus Selector22/1
  HWALineCalc/25(LockID) -> Terminator29/1, Unit Delay65/1  "LSM_LockID"
  Unit Delay65/1 -> HWALineCalc/33(LockIDK1)
  Unit Delay64/1 -> HWALineCalc/34(Lock_counterK1)
  HWALineCalc/26(Lock_counter) -> Terminator30/1, Unit Delay64/1  "LSM_LockCounter"
  Unit Delay63/1 -> VisLineFilter4/23(Avail_timeK1)
  Unit Delay62/1 -> VisLineFilter4/24(Avail_disK1)
  VisLineFilter4/10(Avail_dis) -> Unit Delay62/1, Bus Creator/10
  VisLineFilter4/9(Avail_time) -> Unit Delay63/1, Bus Creator/9
  RFM_LINE_EXIT_CL1/1 -> Bus Selector19/1
  Bus Selector19/1 -> Signal Copy17/1  "<bIsLineExist>"
  Signal Copy17/1 -> Terminator13/1  "LSM_Exit_Valid"
  Bus Selector19/4 -> Signal Copy20/1  "<dC2V>"
  Bus Selector19/3 -> Signal Copy19/1  "<dC1V>"
  Bus Selector19/2 -> Signal Copy18/1  "<dC0V>"
  Bus Selector19/5 -> Signal Copy21/1  "<dC3V>"
  Bus Selector19/6 -> Signal Copy22/1  "<dDisStart>"
  Bus Selector19/7 -> Signal Copy23/1  "<dDisFront>"
  Signal Copy18/1 -> Terminator17/1  "LSM_Exit_C0"
  Signal Copy19/1 -> Terminator18/1  "LSM_Exit_C1"
  Signal Copy20/1 -> Terminator19/1  "LSM_Exit_C2"
  Signal Copy21/1 -> Terminator14/1  "LSM_Exit_C3"
  Signal Copy22/1 -> Terminator15/1  "LSM_Exit_Start"
  Signal Copy23/1 -> Terminator16/1  "LSM_Exit_Front"
  Signal Copy16/1 -> Terminator12/1  "LSM_EN_Front"
  Signal Copy15/1 -> Terminator11/1  "LSM_EN_Start"
  Signal Copy14/1 -> Terminator10/1  "LSM_EN_C3"
  Signal Copy13/1 -> Terminator9/1  "LSM_EN_C2"
  Signal Copy12/1 -> Terminator8/1  "LSM_EN_C1"
  Signal Copy11/1 -> Terminator7/1  "LSM_EN_C0"
  Bus Selector18/7 -> Signal Copy16/1  "<dDisFront>"
  Bus Selector18/6 -> Signal Copy15/1  "<dDisStart>"
  Bus Selector18/5 -> Signal Copy14/1  "<dC3V>"
  Bus Selector18/2 -> Signal Copy11/1  "<dC0V>"
  Bus Selector18/3 -> Signal Copy12/1  "<dC1V>"
  Bus Selector18/4 -> Signal Copy13/1  "<dC2V>"
  Signal Copy10/1 -> Terminator1/1  "LSM_EN_Valid"
  Bus Selector18/1 -> Signal Copy10/1  "<bIsLineExist>"
  Subsystem3/5(LSM_PilotSPL) -> PilotSPL/1  "LSM_PilotSPL"
  Subsystem3/6(PilotSPLDist) -> PilotSPLDist/1  "LSM_PilotSPLDist"
  RFM_LINE_EXIT_CL/1 -> Bus Selector17/1
  RFM_LINE_ENTRY_CL/1 -> Bus Selector18/1
  [PilotSts] -> Compare To Constant3/1
  Mux14/1 -> [VisLineType]
  RightLineType1/1 -> Mux14/2
  LeftLineType1/1 -> Mux14/1
  Signal Copy8/1 -> MLeLane/1, Subsystem3/16(VehInLeftmostLane)  "LSM_LeftMostLane"
  [VisLineConf] -> VehStation/1(VisLineConf)
  [VisLineType] -> VehStation/3(VisLineType)
  [VisEdgeConf] -> VehStation/4(VisEdgeConf)
  [VisLineA0] -> VehStation/2(VisLineA0)
  [VisEdgeA0] -> VehStation/5(VisEdgeA0)
  Subsystem3/3(PilotSts) -> Switch4/3  "LSM_PilotSts"
  Subsystem3/2(PilotTurnSwSts) -> PilotTurnSwSts/1  "LSM_PilotTurnSwSts"
  Subsystem3/1(PilotRoadSts) -> [PilotRoadSts], PilotRoadSts/1  "LSM_PilotRoadSts"
  Bus Selector12/4 -> Signal Copy3/1  "<en_direction>"
  Bus Selector12/2 -> Signal Copy2/1  "<f_start_distance>"
  Bus Selector12/1 -> Signal Copy1/1  "<b_is_available>"
  RFM_ROAD/1 -> Bus Selector13/1
  RFM_INTERSEC_ALERT/1 -> Bus Selector12/1
  Constant14/1 -> VisLineFilter2/17(Lowlimit)
  Unit Delay61/1 -> VisLineFilter2/29(Avail_timeK1)
  VisLineFilter2/12(Avail_time) -> Unit Delay61/1, Bus Creator1/9
  Unit Delay60/1 -> VisLineFilter2/30(Avail_disK1)
  VisLineFilter2/13(Avail_dis) -> Unit Delay60/1, Bus Creator1/10
  TJA2NOA/6(HWARange) -> Bus Creator2/6
  TJA2NOA/5(HWALineC0) -> Bus Creator2/5, Unit Delay49/1
  TJA2NOA/4(HWALineC1) -> Bus Creator2/4
  TJA2NOA/3(HWALineC2) -> Bus Creator2/3
  TJA2NOA/2(HWALineC3) -> Bus Creator2/2
  TJA2NOA/1(HWALineValid) -> Bus Creator2/1
  LineSelect/6(TJALineRange) -> TJA2NOA/6(TJALineRange)  "TJALineRange"
  LineSelect/5(TJALineA0) -> TJA2NOA/5(TJALineA0)  "TJALineA0"
  LineSelect/4(TJALineA1) -> TJA2NOA/4(TJALineA1)  "TJALineA1"
  LineSelect/3(TJALineA2) -> TJA2NOA/3(TJALineA2)  "TJALineA2"
  LineSelect/2(TJALineA3) -> TJA2NOA/2(TJALineA3)  "TJALineA3"
  LineSelect/1(TJALineValid) -> TJA2NOA/1(TJALineValid)  "TJALineValid"
  Bus Selector10/4 -> HWALineA1/1  "<HWALineC1>"
  HWALineCalc/4(HWALineC1) -> Bus Creator4/4
  Bus Selector10/5 -> HWALineA0/1  "<HWALineC0>"
  HWALineCalc/7(HWALeLineValid) -> Bus Creator3/1
  HWALineCalc/11(HWALeLineC0) -> Bus Creator3/5
  HWALineCalc/10(HWALeLineC1) -> Bus Creator3/4
  HWALineCalc/8(HWALeLineC3) -> Bus Creator3/2
  Bus Selector9/6 -> TJALineRange/1  "<HWARange>"
  Switch1/1 -> Bus Selector9/1
  Bus Creator2/1 -> Switch1/3, [TJA_Line]
  Switch/1 -> Bus Selector10/1, Bus Selector39/1
  Bus Selector9/5 -> TJALineA0/1  "<HWALineC0>"
  Bus Selector9/3 -> TJALineA2/1  "<HWALineC2>"
  Bus Selector9/4 -> TJALineA1/1  "<HWALineC1>"
  Bus Selector10/3 -> HWALineA2/1  "<HWALineC2>"
  Bus Selector9/1 -> TJALineValid/1  "<HWALineValid>"
  HWALineCalc/1(HWALineValid) -> Bus Creator4/1
  Bus Selector10/6 -> HWALineRange/1  "<HWARange>"
  HWALineCalc/5(HWALineC0) -> Bus Creator4/5, [HWALineC0]
  HWALineCalc/12(HWALeRange) -> Bus Creator3/6
  Bus Selector9/2 -> TJALineA3/1  "<HWALineC3>"
  Bus Selector10/2 -> HWALineA3/1  "<HWALineC3>"
  HWALineCalc/9(HWALeLineC2) -> Bus Creator3/3
  Bus Creator4/1 -> Switch/3
  HWALineCalc/2(HWALineC3) -> Bus Creator4/2
  Bus Selector10/1 -> HWALineValid/1  "<HWALineValid>"
  Bus Selector11/6 -> MATLAB Function1/14(LeLineRange)  "<HWALeRange>"
  Bus Selector11/4 -> MATLAB Function1/12(LeLineC1)  "<HWALeLineC1>"
  Bus Selector11/3 -> MATLAB Function1/11(LeLineC2)  "<HWALeLineC2>"
  Bus Selector11/1 -> MATLAB Function1/9(LeLineValid)  "<HWALeLineValid>"
  Switch2/1 -> Bus Selector11/1
  Bus Creator3/1 -> Switch2/3
  Bus Selector11/2 -> MATLAB Function1/10(LeLineC3)  "<HWALeLineC3>"
  Bus Selector11/5 -> MATLAB Function1/13(LeLineC0)  "<HWALeLineC0>"
  HWALineCalc/6(HWARange) -> Bus Creator4/6
  HWALineCalc/3(HWALineC2) -> Bus Creator4/3
  AND1/1 -> Switch/2, Switch2/2, Switch3/2
  Bus Selector4/5 -> ESSLineCalc1/16(EdgeA0)  "<EdgeA0>"
  Bus Selector4/4 -> ESSLineCalc1/15(EdgeA1)  "<EdgeA1>"
  Bus Selector3/7 -> ESSLineCalc1/11(tLost)  "<tLost>"
  Bus Selector3/6 -> ESSLineCalc1/10(Range)  "<Range>"
  Bus Selector3/5 -> ESSLineCalc1/9(A0)  "<A0>"
  Bus Selector3/4 -> ESSLineCalc1/8(A1)  "<A1>"
  Bus Selector2/8 -> HWALineCalc/16(tLost)  "<tLost>"
  Bus Selector2/7 -> HWALineCalc/15(Range)  "<Range>"
  Bus Selector2/6 -> HWALineCalc/14(A0)  "<A0>"
  Bus Selector2/5 -> HWALineCalc/13(A1)  "<A1>"
  Bus Selector2/4 -> HWALineCalc/12(A2)  "<A2>"
  Bus Selector2/3 -> HWALineCalc/11(A3)  "<A3>"
  Bus Selector2/1 -> HWALineCalc/9(LineConf)  "<LineConf>"
  Bus Selector5/3 -> LREWidthCalc/3(a0)  "<EdgeA0>"
  Bus Selector5/2 -> LREWidthCalc/2(a1)  "<EdgeA1>"
  Bus Selector/3 -> RoadWidthCalc1/4(a0)  "<A0>"
  Bus Selector/2 -> RoadWidthCalc1/3(a1)  "<A1>"
  [VisEdge] -> CenLineCal1/5(VisEdge)
  [VisLine] -> CenLineCal1/4(VisLine)
  VisLineFilter4/8(EdgetLost) -> Bus Creator/8, Unit Delay17/1
  Unit Delay38/1 -> VisLineFilter4/16(EdgeReliableK1)
  VisLineFilter4/2(EdgeReliable) -> Bus Creator/2, Unit Delay38/1
  [VisEdgeReliable] -> VisLineFilter4/3(VisEdgeReliable)
  Unit Delay37/1 -> VisLineFilter2/22(LineReliableK1)
  VisLineFilter2/5(LineReliable) -> Bus Creator1/2, Unit Delay37/1
  [VisLineReliable] -> VisLineFilter2/5(VisLineReliable)
  Mux13/1 -> [VisEdgeReliable]
  Edge2_Re/1 -> Mux13/2
  Edge1_Re/1 -> Mux13/1
  Mux12/1 -> [VisLineReliable]
  L1_Re/1 -> Mux12/1
  L2_Re/1 -> Mux12/2
  L3_Re/1 -> Mux12/3
  L4_Re/1 -> Mux12/4
  LREWidthCalc/1(LREWidth) -> Unit Delay36/1, [LREWidth]
  [VisEdgeUpdate] -> LREWidthCalc/4(LRELineUpdate)
  [VisEdge] -> Bus Selector5/1
  Unit Delay36/1 -> LREWidthCalc/5(LREWidthK1)
  Bus Selector5/1 -> LREWidthCalc/1(LRELineConf)  "<EdgeConf>"
  RightDLM/1 -> TypeConf/5(RightDLMType)
  LeftDLM/1 -> TypeConf/2(LeftDLMType)
  Bus Selector6/6 -> LineSelect/6(CentRange)  "<CentLineRange>"
  Bus Selector6/5 -> LineSelect/5(CentLineA0)  "<CentLineC0>"
  Bus Selector6/4 -> LineSelect/4(CentLineA1)  "<CentLineC1>"
  Bus Selector6/3 -> LineSelect/3(CentLineA2)  "<CentLineC2>"
  Bus Selector6/2 -> LineSelect/2(CentLineA3)  "<CentLineC3>"
  Bus Selector6/1 -> LineSelect/1(CentLaneValid)  "<CentLineConf>"
  CenLineCal1/1(CenLine) -> [CentLine], Bus Selector6/1
  kap/1 -> CalcEgoVehMove/2(Kap)
  vRef1/1 -> CalcEgoVehMove/3(Vego)
  CalcEgoVehMove/2(dDeltaY) -> [dDeltaY]
  CalcEgoVehMove/4(SinOfPsi) -> [SinOfPsi]
  CalcEgoVehMove/3(CosOfPsi) -> [CosOfPsi]
  CalcEgoVehMove/1(dDeltaX) -> [dDeltaX]
  Constant/1 -> CalcEgoVehMove/1(tCycle)
  CalcEgoVehMove2/1(dDeltaX) -> HWALineCalc/26(dDeltaX)
  [VisLineA0] -> YBranchRi/8(A0)
  Unit Delay32/1 -> YBranchRi/11(DistK1)
  HWALineCalc/24(MoveID) -> Terminator28/1, Unit Delay30/1  "LSM_MoveID"
  [VisLineUpdate] -> YBranchRi/1(LineUpdate)
  LeftLineType/1 -> Compare To Constant59/1, TypeConf/1(LeftType)
  [VisLine] -> Bus Selector/1
  HWALineCalc/13(HWARiLineValid) -> Bus Creator7/1
  [RightOffset_b] -> YBranchRi/2(RightOffset_b)
  Bus Selector1/1 -> Selector1/1  "<LineConf>"
  TypeConf/2(Out2) -> HWALineCalc/2(RightLineTypeEn), [RightLineTypeEN]
  HWALineCalc/14(HWARiLineC3) -> Bus Creator7/2
  Unit Delay14/1 -> RoadWidthCalc1/6(RoadWidthK1)
  HWASts/1 -> HWALineCalc/7(HWASts), Unit Delay16/1
  CalcEgoVehMove2/4(SinOfPsi) -> HWALineCalc/29(SinOfPsi)
  kap4/1 -> CalcEgoVehMove2/2(Kap)
  [VisLineA3] -> YBranchRi/5(A3)
  Constant7/1 -> CalcEgoVehMove2/1(tCycle)
  HWALineCalc/23(DoubleLineLost_b) -> Terminator41/1
  Unit Delay33/1 -> YBranchRi/4(RoadWidth)
  TrueDurationTime/1 -> Compare To Constant60/1
  CalcEgoVehMove2/3(CosOfPsi) -> HWALineCalc/28(CosOfPsi)
  Unit Delay15/1 -> RoadWidthCalc1/7(tLostK1)
  vRef5/1 -> Compare To Zero/1
  Unit Delay16/1 -> HWALineCalc/8(HWAStsK1)
  HWALineCalc/20(HeadAngDiff) -> pre_HeadAng_Error/1
  vRef7/1 -> CalcEgoVehMove2/3(Vego), D/1, HWALineCalc/30(vRef)
  Selector1/1 -> Compare To Constant1/1
  Compare To Zero/1 -> Logical Operator/3
  CalcEgoVehMove2/2(dDeltaY) -> HWALineCalc/27(dDeltaY)
  HWALineCalc/16(HWARiLineC1) -> Bus Creator7/4
  [LeftOffset_b] -> HWALineCalc/23(LeftOffset_b)
  [VisLine] -> Bus Selector2/1
  Unit Delay30/1 -> HWALineCalc/32(MoveIDK1)
  RightLineType/1 -> TypeConf/4(RightType)
  [RightOffset_b] -> HWALineCalc/24(RightOffset_b)
  [RoadWidth] -> HWALineCalc/25(RoadWidth)
  [VisLineA1] -> YBranchRi/7(A1)
  [VisLineUpdate] -> RoadWidthCalc1/5(LineUpdate)
  RoadWidthCalc1/1(RoadWidth) -> [RoadWidth], Unit Delay14/1, RoadWidth/1
  RoadWidthCalc1/2(tLost) -> Unit Delay15/1
  HWALineCalc/21(Error) -> Terminator/1
  HWALineCalc/15(HWARiLineC2) -> Bus Creator7/3
  HWALineCalc/22(SingleLineLost_b) -> SingleLineLost_b/1
  vRef12/1 -> YBranchRi/3(vRef)
  YBranchRi/3(Dist) -> Unit Delay32/1
  HWALineCalc/19(preDyDiff) -> pre_dy_Error/1
  [RoadWidth] -> Unit Delay33/1
  HWALineCalc/17(HWARiLineC0) -> Bus Creator7/5
  TypeConf/1(Out1) -> [LeftLineTypeEN], HWALineCalc/1(LeftLineTypeEn)
  [VisLineA2] -> YBranchRi/6(A2)
  Compare To Constant59/1 -> Logical Operator/2
  Logical Operator/1 -> TrueDurationTime/1
  Compare To Constant60/1 -> leftLaneCurise_b/1  "leftLaneCurise_b"
  YBranchRi/2(YBranchRi_b) -> HWALineCalc/4(YBranchRi_b)
  YBranchRi/4(DistRi) -> Unit Delay34/1
  Compare To Constant1/1 -> Logical Operator/1
  Unit Delay34/1 -> YBranchRi/12(DistRiK1)
  [VisLine] -> Bus Selector1/1
  HWALineCalc/18(HWARiRange) -> Bus Creator7/6
  [VisLineConf] -> YBranchRi/9(Conf)
  Bus Selector/1 -> RoadWidthCalc1/2(VisLineConf)  "<LineConf>"
  D/1 -> HWALineCalc/31(DistanceLim)
  YBranchRi/1(YBranch_b) -> HWALineCalc/3(YBranch_b), RoadWidthCalc1/1(YBranch_b)
  DetectIncrease1/1(out) -> VisLineFilter2/20(RightLineChange), [RiLineCrossing], [RightOffset_b]
  Tracker/2(RightOffset_b) -> Logical Operator2/1
  RightLine_Change/1 -> Logical Operator2/2
  Tracker/1(LeftOffset_b) -> Logical Operator1/2
  LeftLine_Change/1 -> Logical Operator1/1
  kap3/1 -> CalcEgoVehMove1/2(Kap)
  [VisLineA2] -> VisLineFilter2/7(a2)
  Unit Delay4/1 -> VisLineFilter2/27(RangeK1)
  Unit Delay2/1 -> VisLineFilter2/28(tLostK1)
  Tracker/8(pre_A0_2) -> Unit Delay11/1
  CalcEgoVehMove1/1(dDeltaX) -> Tracker/7(dDeltaX)
  Tracker/4(error_left) -> Terminator3/1
  VisLineFilter2/4(LineConf) -> Bus Creator1/1, Unit Delay57/1
  Tracker/3(error_right) -> Terminator2/1
  CalcEgoVehMove1/3(CosOfPsi) -> Tracker/9(CosOfPsi)
  vRef4/1 -> CalcEgoVehMove1/3(Vego)
  Unit Delay13/1 -> Tracker/13(pre_A2_2K1)
  Tracker/7(pre_A1_2) -> Unit Delay12/1
  Tracker/10(pre_A2_3) -> Unit Delay59/1
  [dDeltaY] -> VisLineFilter2/13(dDeltaY)
  Tracker/9(pre_A3_3) -> Unit Delay10/1
  Unit Delay58/1 -> Tracker/18(pre_A1_3K1)
  Unit Delay1/1 -> Tracker/19(pre_A0_3K1)
  Unit Delay3/1 -> VisLineFilter2/18(RoadWidth)
  [VisLineA0] -> VisLineFilter2/9(a0)
  Unit Delay6/1 -> Tracker/12(pre_A3_2K1)
  Bus Creator1/1 -> [VisLine]
  VisLineFilter2/9(A0) -> Bus Creator1/6, Unit Delay5/1
  Tracker/13(pre_LineConf) -> Unit Delay35/1
  Unit Delay35/1 -> Tracker/20(pre_LineConfK1)
  vRef9/1 -> Tracker/11(vRef)
  Unit Delay5/1 -> VisLineFilter2/26(A0K1)
  Unit Delay10/1 -> Tracker/16(pre_A3_3K1)
  VisLineFilter2/1(DevValid) -> Terminator4/1
  Tracker/6(pre_A2_2) -> Unit Delay13/1
  Unit Delay11/1 -> Tracker/15(pre_A0_2K1)
  [VisLineConf] -> VisLineFilter2/4(VisLineConf)
  Unit Delay12/1 -> Tracker/14(pre_A1_2K1)
  [VisLineR] -> VisLineFilter2/10(R)
  Unit Delay7/1 -> VisLineFilter2/25(A1K1)
  Unit Delay9/1 -> VisLineFilter2/23(A3K1)
  Unit Delay8/1 -> VisLineFilter2/24(A2K1)
  [dDeltaX] -> VisLineFilter2/12(dDeltaX)
  Unit Delay57/1 -> VisLineFilter2/21(LineConfK1)
  [VisLineUpdate] -> Tracker/1(LineUpdate)
  VisLineFilter2/10(Range) -> Bus Creator1/7, Unit Delay4/1
  tFilt/1 -> VisLineFilter2/2(tF)
  [VisLineA1] -> VisLineFilter2/8(a1)
  VisLineFilter2/2(DevAngle) -> Terminator5/1
  CalcEgoVehMove1/4(SinOfPsi) -> Tracker/10(SinOfPsi)
  [RoadWidth] -> Unit Delay3/1
  [VisLineA3] -> Tracker/6(A3)
  [VisLineA0] -> Tracker/3(A0)
  CalcEgoVehMove1/2(dDeltaY) -> Tracker/8(dDeltaY)
  Constant3/1 -> VisLineFilter2/3(tCycle)
  [VisLineUpdate] -> VisLineFilter2/11(LineUpdate)
  VisLineFilter2/3(DevDis) -> Terminator6/1
  Unit Delay59/1 -> Tracker/17(pre_A2_3K1)
  [VisLineConf] -> Tracker/2(LineConf)
  Constant6/1 -> CalcEgoVehMove1/1(tCycle)
  [SinOfPsi] -> VisLineFilter2/15(SinOfPsi)
  [VisLineA2] -> Tracker/5(A2)
  VisLineFilter2/11(tLost) -> Bus Creator1/8, Unit Delay2/1
  [CosOfPsi] -> VisLineFilter2/14(CosOfPsi)
  VisLineFilter2/7(A2) -> Bus Creator1/4, Unit Delay8/1
  Tracker/5(pre_A3_2) -> Unit Delay6/1
  VisLineFilter2/6(A3) -> Bus Creator1/3, Unit Delay9/1
  VisLineFilter2/8(A1) -> Bus Creator1/5, Unit Delay7/1
  [VisLineA3] -> VisLineFilter2/6(a3)
  vRef/1 -> VisLineFilter2/16(vRef)
  Tracker/12(pre_A0_3) -> Unit Delay1/1
  [VisLineA1] -> Tracker/4(A1)
  Tracker/11(pre_A1_3) -> Unit Delay58/1
  Unit Delay24/1 -> ESSLineCalc1/4(ESSStsK1)
  Data Type Conversion1/1 -> ESSLineCalc1/12(EdgeValid)
  ESSLineCalc1/18(ESSRiRange) -> ESSLineRRange/1
  ESSLineCalc1/13(ESSRiLineValid) -> ESSLineRValid/1
  ESSLineCalc1/12(ESSLeRange) -> ESSLineLRange/1
  ESSLineCalc1/10(ESSLeLineA1) -> ESSLineLA1/1
  ESSLineCalc1/9(ESSLeLineA2) -> ESSLineLA2/1
  ESSLineCalc1/8(ESSLeLineA3) -> ESSLineLA3/1
  ESSLineCalc1/5(ESSLineA0) -> ESSLineA0/1
  ESSLineCalc1/4(ESSLineA1) -> ESSLineA1/1
  ESSLineCalc1/3(ESSLineA2) -> ESSLineA2/1
  ESSLineCalc1/2(ESSLineA3) -> ESSLineA3/1
  ESSLineCalc1/7(ESSLeLineValid) -> ESSLineLValid/1
  ESSLineCalc1/6(ESSRange) -> ESSLineRange/1
  ESSLineCalc1/1(ESSLineValid) -> ESSLineValid/1
  ESSLineCalc1/11(ESSLeLineA0) -> ESSLineLA0/1
  ESSLineCalc1/14(ESSRiLineA3) -> ESSLineRA3/1
  ESSLineCalc1/15(ESSRiLineA2) -> ESSLineRA2/1
  ESSLineCalc1/16(ESSRiLineA1) -> ESSLineRA1/1
  ESSLineCalc1/17(ESSRiLineA0) -> ESSLineRA0/1
  Unit Delay26/1 -> ESSLineCalc1/21(MoveIDK1)
  ESSLineCalc1/19(MoveID) -> Unit Delay26/1
  Unit Delay25/1 -> ESSLineCalc1/22(Lock_bK1)
  ESSLineCalc1/20(Lock_b) -> Unit Delay25/1, ESSLineLock_b/1
  D1/1 -> ESSLineCalc1/20(ESSDistLim)
  vRef3/1 -> D1/1
  [RoadWidth] -> ESSLineCalc1/19(RoadWidth)
  [RightOffset_b] -> ESSLineCalc1/18(RightOffset_b)
  [LeftOffset_b] -> ESSLineCalc1/17(LeftOffset_b)
  Bus Selector4/3 -> ESSLineCalc1/14(EdgeA2)  "<EdgeA2>"
  Bus Selector4/1 -> Data Type Conversion1/1  "<EdgeConf>"
  Bus Selector4/2 -> ESSLineCalc1/13(EdgeA3)  "<EdgeA3>"
  [VisEdge] -> Bus Selector4/1
  Bus Selector3/1 -> ESSLineCalc1/5(LineConf)  "<LineConf>"
  Bus Selector3/2 -> ESSLineCalc1/6(A3)  "<A3>"
  Bus Selector3/3 -> ESSLineCalc1/7(A2)  "<A2>"
  [VisLine] -> Bus Selector3/1
  ESSSts/1 -> Unit Delay24/1, ESSLineCalc1/3(ESSSts)
  Bus Creator/1 -> [VisEdge]
  DetectChange/1(Out1) -> VisLineFilter1/9(LineUpdate)
  OTLCount/1 -> DetectChange/1(OTLCount)
  OTLineValid/1 -> VisLineFilter1/3(OTLineValid)
  Edge1_Conf/1 -> Mux11/1
  Edge2_Conf/1 -> Mux11/2
  Mux11/1 -> [VisEdgeConf]
  Mux10/1 -> [VisEdgeA0]
  Edge2_A0/1 -> Mux10/2
  Edge1_A0/1 -> Mux10/1
  Edge1_A1/1 -> Mux9/1
  Edge2_A1/1 -> Mux9/2
  Mux9/1 -> [VisEdgeA1]
  Mux8/1 -> [VisEdgeA2]
  Edge2_A2/1 -> Mux8/2
  Edge1_A2/1 -> Mux8/1
  Mux7/1 -> [VisEdgeA3]
  Edge1_A3/1 -> Mux7/1
  Edge2_A3/1 -> Mux7/2
  Edge2_R/1 -> Mux6/2
  Edge1_R/1 -> Mux6/1
  Mux6/1 -> [VisEdgeRange]
  LRELineUpdate/1 -> [VisEdgeUpdate]
  LALineUpdate/1 -> [VisLineUpdate]
  L4_R/1 -> Mux5/4
  L3_R/1 -> Mux5/3
  L2_R/1 -> Mux5/2
  L1_R/1 -> Mux5/1
  L4_A0/1 -> Mux4/4
  L3_A0/1 -> Mux4/3
  L2_A0/1 -> Mux4/2
  L1_A0/1 -> Mux4/1
  Mux5/1 -> [VisLineR]
  Mux4/1 -> [VisLineA0]
  L4_A1/1 -> Mux3/4
  L3_A1/1 -> Mux3/3
  L2_A1/1 -> Mux3/2
  L1_A1/1 -> Mux3/1
  Mux3/1 -> [VisLineA1]
  Mux2/1 -> [VisLineA2]
  L4_A2/1 -> Mux2/4
  L3_A2/1 -> Mux2/3
  L2_A2/1 -> Mux2/2
  L1_A2/1 -> Mux2/1
  L4_A3/1 -> Mux1/4
  L3_A3/1 -> Mux1/3
  L2_A3/1 -> Mux1/2
  L1_A3/1 -> Mux1/1
  L4_Conf/1 -> Mux/4
  L3_Conf/1 -> Mux/3
  L2_Conf/1 -> Mux/2
  L1_Conf/1 -> Mux/1
  vRef6/1 -> VisLineFilter4/14(vRef)
  [SinOfPsi] -> VisLineFilter4/13(SinOfPsi)
  [CosOfPsi] -> VisLineFilter4/12(CosOfPsi)
  [dDeltaY] -> VisLineFilter4/11(dDeltaY)
  [dDeltaX] -> VisLineFilter4/10(dDeltaX)
  [VisEdgeUpdate] -> VisLineFilter4/9(LineUpdate)
  [VisEdgeRange] -> VisLineFilter4/8(R)
  [VisEdgeA0] -> VisLineFilter4/7(a0)
  [VisEdgeA1] -> VisLineFilter4/6(a1)
  [VisEdgeA2] -> VisLineFilter4/5(a2)
  [VisEdgeA3] -> VisLineFilter4/4(a3)
  Constant4/1 -> VisLineFilter4/1(tCycle)
  [VisEdgeConf] -> VisLineFilter4/2(VisEdgeConf)
  Unit Delay17/1 -> VisLineFilter4/22(EdgetLostK1)
  VisLineFilter4/7(EdgeRange) -> Unit Delay18/1, Bus Creator/7
  Unit Delay18/1 -> VisLineFilter4/21(EdgeRangeK1)
  VisLineFilter4/6(EdgeA0) -> Unit Delay19/1, Bus Creator/6
  Unit Delay19/1 -> VisLineFilter4/20(EdgeA0K1)
  VisLineFilter4/5(EdgeA1) -> Unit Delay20/1, Bus Creator/5
  Unit Delay20/1 -> VisLineFilter4/19(EdgeA1K1)
  VisLineFilter4/4(EdgeA2) -> Unit Delay21/1, Bus Creator/4
  VisLineFilter4/3(EdgeA3) -> Bus Creator/3, Unit Delay22/1
  VisLineFilter4/1(EdgeConf) -> Bus Creator/1, Unit Delay23/1
  Unit Delay21/1 -> VisLineFilter4/18(EdgeA2K1)
  Unit Delay22/1 -> VisLineFilter4/17(EdgeA3K1)
  Unit Delay23/1 -> VisLineFilter4/15(EdgeConfK1)
  Mux/1 -> [VisLineConf]
  Mux1/1 -> [VisLineA3]
  [SinOfPsi] -> VisLineFilter1/13(SinOfPsi)
  [CosOfPsi] -> VisLineFilter1/12(CosOfPsi)
  [dDeltaY] -> VisLineFilter1/11(dDeltaY)
  [dDeltaX] -> VisLineFilter1/10(dDeltaX)
  LineSelect/7(LCKLineValid) -> LCKLineValid/1
  LineSelect/8(LCKLineA3) -> LCKLineA3/1
  LineSelect/9(LCKLineA2) -> LCKLineA2/1
  LineSelect/10(LCKLineA1) -> LCKLineA1/1
  LineSelect/11(LCKLineA0) -> LCKLineA0/1
  LineSelect/12(LCKLineRange) -> LCKLineRange/1
  dxMax/1 -> VisLineFilter1/8(R)
  aOTL/1 -> VisLineFilter1/4(aOTL)
  Constant2/1 -> VisLineFilter1/1(tCycle)
  VisLineFilter1/2(A3) -> Unit Delay43/1, Subsystem2/5(DOP_C3)
  Unit Delay45/1 -> VisLineFilter1/19(RangeK1)
  Unit Delay43/1 -> VisLineFilter1/15(A3K1)
  VisLineFilter1/1(LineValid) -> Subsystem2/4(DOP_Valid), Unit Delay42/1
  Unit Delay48/1 -> VisLineFilter1/16(A2K1)
  Unit Delay42/1 -> VisLineFilter1/14(LineValidK1)
  Unit Delay47/1 -> VisLineFilter1/17(A1K1)
  Unit Delay44/1 -> VisLineFilter1/20(tLostK1)
  VisLineFilter1/6(Range) -> Unit Delay45/1, Subsystem2/9(DOP_Range)
  VisLineFilter1/7(tLost) -> Unit Delay44/1
  Unit Delay46/1 -> VisLineFilter1/18(A0K1)
  VisLineFilter1/4(A1) -> Unit Delay47/1, Subsystem2/7(DOP_C1)
  VisLineFilter1/5(A0) -> Unit Delay46/1, Subsystem2/8(DOP_C0)
  VisLineFilter1/3(A2) -> Unit Delay48/1, Subsystem2/6(DOP_C2)
  ACCmode/1 -> Terminator35/1
  Signal Copy1/1 -> Subsystem3/1(Intersec_available)
  Signal Copy2/1 -> Subsystem3/2(f_distance)
  Signal Copy3/1 -> Subsystem3/4(en_direction)
  Signal Copy4/1 -> Subsystem3/5(i_rec_lanes_num)
  Signal Copy5/1 -> Subsystem3/6(i_rec_lanes)
  Signal Copy6/1 -> Subsystem3/7(nLaneNum)
  Signal Copy7/1 -> Subsystem3/8(nLaneID)
  Signal Copy9/1 -> Subsystem3/9(i_mapvalid)
  Signal Copy36/1 -> Subsystem3/10(i_on_nav_path)
  Signal Copy37/1 -> Data Type Conversion/1
  Signal Copy39/1 -> Subsystem3/12(Exit_dDisStart)
  Signal Copy40/1 -> Subsystem3/13(ExitLineExist)
  Signal Copy41/1 -> Subsystem3/14(Exit_dC0V)
  Signal Copy42/1 -> Subsystem3/15(RoadType)
  Signal Copy44/1 -> Subsystem3/18(Entry_bIsLineExist)
  Signal Copy45/1 -> Subsystem3/19(Entry_dDisStart)
  Signal Copy46/1 -> Subsystem3/20(Entry_dC0V)
  Signal Copy47/1 -> Subsystem3/21("curr_f_vanish_pt_dis ")
  Signal Copy48/1 -> Subsystem3/22(currentLane_type)
  Signal Copy49/1 -> Subsystem3/26(rightLane_valid)
  Signal Copy50/1 -> Subsystem3/27(rightLane_type)
  Signal Copy51/1 -> Subsystem3/30(leftLane_valid)
  Signal Copy52/1 -> Subsystem3/31(leftLane_type)
  Signal Copy53/1 -> Subsystem3/34(RFM_ODD)
  [PilotSts] -> Compare To Constant13/1
  Compare To Constant14/1 -> AND2/1
  NOH_Sts1/1 -> Compare To Constant14/1
  Compare To Constant13/1 -> AND2/2
  AND2/1 -> Switch8/2, Switch7/2
  [RiLineCrossing] -> Switch7/3
  [LeLineCrossing] -> Switch8/3
  Switch7/1 -> RiLineCrossing/1
  [SPL_LaneChanged] -> Compare To Constant15/1
  Compare To Constant15/1 -> Switch7/1
  Switch8/1 -> LeLineCrossing/1
  Compare To Constant16/1 -> Switch8/1
  [SPL_LaneChanged] -> Compare To Constant16/1
  HWASts2/1 -> MATLAB Function1/1(HWASts)
  [RoadWidth] -> MATLAB Function1/2(RoadWidth)
  Bus Selector39/2 -> MATLAB Function1/4(LineC3)  "<HWALineC3>"
  Bus Selector39/1 -> MATLAB Function1/3(LineValid)  "<HWALineValid>"
  Bus Selector39/3 -> MATLAB Function1/5(LineC2)  "<HWALineC2>"
  Bus Selector39/4 -> MATLAB Function1/6(LineC1)  "<HWALineC1>"
  Bus Selector39/5 -> MATLAB Function1/7(LineC0)  "<HWALineC0>"
  Bus Selector39/6 -> MATLAB Function1/8(LineRange)  "<HWARange>"
  MATLAB Function1/7(LeLineVirtual_b) -> LeLineVirtual_b/1
  MATLAB Function1/14(RiLineVirtual_b) -> RiLineVirtual_b/1
  MATLAB Function1/1(HWALeLineValid) -> HWALineLValid/1
  MATLAB Function1/2(HWALeLineC3) -> HWALineLA3/1
  MATLAB Function1/3(HWALeLineC2) -> HWALineLA2/1
  MATLAB Function1/4(HWALeLineC1) -> HWALineLA1/1
  MATLAB Function1/5(HWALeLineC0) -> HWALineLA0/1
  MATLAB Function1/6(HWALeLineRange) -> HWALineLRange/1
  MATLAB Function1/8(HWARiLineValid) -> HWALineRValid/1
  MATLAB Function1/9(HWARiLineC3) -> HWALineRA3/1
  MATLAB Function1/10(HWARiLineC2) -> HWALineRA2/1
  MATLAB Function1/11(HWARiLineC1) -> HWALineRA1/1
  MATLAB Function1/12(HWARiLineC0) -> HWALineRA0/1
  MATLAB Function1/13(HWARiLineRange) -> HWALineRRange/1
  Bus Selector25/3 -> Signal Copy54/1  "<b_vanish_valid>"
  Bus Selector25/4 -> Signal Copy55/1  "<f_vanish_pt_dis>"
  Bus Selector38/3 -> Signal Copy56/1  "<b_vanish_valid>"
  Bus Selector38/4 -> Signal Copy57/1  "<f_vanish_pt_dis>"
  Signal Copy54/1 -> Subsystem3/32(left_b_vanish_valid)
  Signal Copy55/1 -> Subsystem3/33(" left_f_vanish_pt_dis")
  Signal Copy56/1 -> Subsystem3/28(right_b_vanish_valid)
  Signal Copy57/1 -> Subsystem3/29(right_f_vanish_pt_dis)
  [PilotSts] -> Compare To Constant17/1
  Compare To Constant17/1 -> AND3/2
  NOH_Sts3/1 -> Compare To Constant18/1
  Compare To Constant18/1 -> AND3/1
  AND3/1 -> Switch9/2
  [RFM_LeLineLcAvailable] -> Bus Creator9/1  "LeftEn"
  [RFM_RiLineLcAvailable] -> Bus Creator9/2  "RightEn"
  Bus Creator9/1 -> Switch9/1
  [LeftLineTypeEN] -> Bus Creator10/1  "LeftEn"
  [RightLineTypeEN] -> Bus Creator10/2  "RightEn"
  Bus Creator10/1 -> Switch9/3
  Switch9/1 -> Bus Selector40/1
  Bus Selector40/1 -> LeLineLcAvailable/1  "<LeftEn>"
  Bus Selector40/2 -> RiLineLcAvailable/1  "<RightEn>"
  Bus Selector12/3 -> Signal Copy38/1  "<f_end_distance>"
  Signal Copy38/1 -> Subsystem3/3(f_end_dis)
  NOH_Sts4/1 -> Subsystem3/35(NOH_Sts)
  Compare To Constant19/1 -> Data Type Conversion9/1
  Data Type Conversion9/1 -> NOA/28(Exit_Valid)
  [preDis] -> NOA/3(preDis)
  [Double_Line_Lost] -> Subsystem3/37(Double_Line_Lost)
